simulink model "test_simulink_model"  (R2019a)
settings: Solver=VariableStepAuto  StartTime=0.0  StopTime=10.0  RelTol=1e-3
settings Model: Creator=marceca  LastModifiedBy=marceca

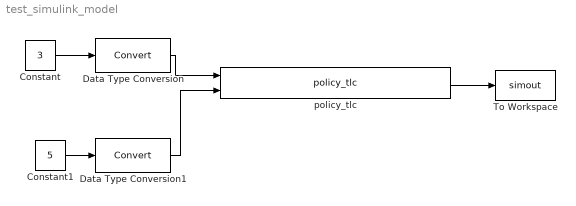
== system test_simulink_model ==
  Constant : Constant  Value=3
  Constant1 : Constant  Value=5
  Data Type Conversion : DataTypeConversion
  Data Type Conversion1 : DataTypeConversion
  To Workspace : ToWorkspace  VariableName=simout  SaveFormat=Timeseries  SampleTime=-1
  policy_tlc : S-Function  FunctionName=policy_tlc  SFunctionDeploymentMode=off  EnableBusSupport=off  mask(Legacy Function){SFunctionSpec=run(int32 u1[1], int32 u2[1], int32 y1[1]), ShowSpec=on}
      mask prompts: ShowSpec "Display function specification"
      mask help:
      | This block allows you to call the legacy functions specified by the following Legacy Code Tool definition:
      | def.SFunctionName = 'policy_tlc';
      | def.OutputFcnSpec = 'run(int32 u1[1], int32 u2[1], int32 y1[1])';
      | def.StartFcnSpec = 'CreateNetwork()';
      | def.TerminateFcnSpec = 'DeleteNetwork()';
      | def.HeaderFiles = {'my_policy_export_toy.h'};
      | def.HostLibFiles = {'libpolicy_export_toy.so'};
      | def.TargetLibFiles = {'libpolicy_export_toy.so'};
      | def.IncPaths = {'inc'};
      | def.LibPaths = {'lib'};
      mask Help: <p>This block was generated automatically by the Legacy Code Tool. For detailed help on this tool, call<a href="matlab:legacy_code('help')"> legacy_code('help')</a>.</p>
      mask Callback ShowSpec:
      | if strcmp(get_param(gcbh, 'ShowSpec'), 'on')
      |   set_param(gcbh, 'MaskDisplay', sprintf('fprintf(''%s'');', get_param(gcbh, 'SFunctionSpec')));
      | else
      |   set_param(gcbh, 'MaskDisplay', sprintf('fprintf(''%s'');', get_param(gcbh, 'FunctionName')));
      | end
      mask Display: fprintf('run(int32 u1[1], int32 u2[1], int32 y1[1])');
  wires:
  Constant/1 -> Data Type Conversion/1
  Constant1/1 -> Data Type Conversion1/1
  policy_tlc/1 -> To Workspace/1
  Data Type Conversion/1 -> policy_tlc/1
  Data Type Conversion1/1 -> policy_tlc/2
